simulink model "week1problem7"  (R2020b)
settings: Solver=VariableStepAuto  StartTime=0.0  StopTime=10.0  RelTol=1e-3
libraries: dspsrcs4 x1
settings Model: Creator=Puru Gawande  LastModifiedBy=Puru Gawande

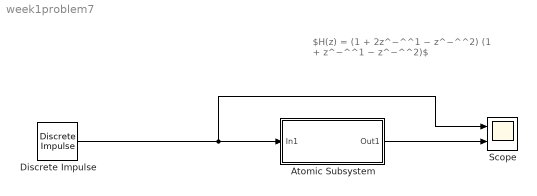
== system week1problem7 ==
  note: $H(z) = (1 + 2z^−^^1 − z^−^^2) (1 + z^−^^1 − z^−^^2)$
  Atomic Subsystem : Subsystem  TreatAsAtomicUnit=on
  Discrete Impulse : dspsrcs4/Discrete  Impulse  Delay=5  SampleTime=0.5  FrameSample=1  OutputFrames=off  dataType=double  isSigned=on  wordLen=16  udDataType=sfix(16)  fracBitsMode=Best precision  numFracBits=15  OutDataTypeStr=double  LastOutDataTypeStr=double
  Scope : Scope  NumInputPorts=2
  wires:
  Discrete Impulse/1 -> Scope/1, Atomic Subsystem/1(In1)
  Atomic Subsystem/1(Out1) -> Scope/2

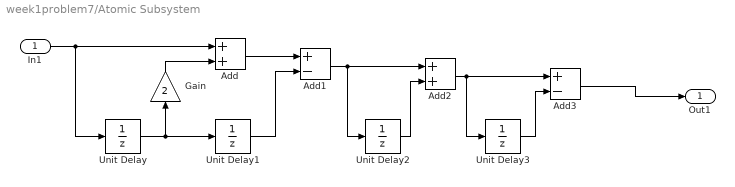
== system week1problem7/Atomic Subsystem ==
  In1 : Inport
  Add : Sum
  Add1 : Sum  Inputs=+-
  Add2 : Sum
  Add3 : Sum  Inputs=+-
  Gain : Gain  Gain=2
  Unit Delay{,1..3} (4 alike) : UnitDelay  SampleTime=-1  HasFrameUpgradeWarning=on
  Out1 : Outport
  wires:
  Unit Delay/1 -> Unit Delay1/1, Gain/1
  Unit Delay2/1 -> Add2/2
  Add1/1 -> Unit Delay2/1, Add2/1
  Unit Delay1/1 -> Add1/2
  In1/1 -> Add/1, Unit Delay/1
  Gain/1 -> Add/2
  Add/1 -> Add1/1
  Unit Delay3/1 -> Add3/2
  Add2/1 -> Unit Delay3/1, Add3/1
  Add3/1 -> Out1/1
